simulink model "LTS_GGV"  (R2024b)
settings: Solver=ode4  StartTime=0.0  StopTime=5  FixedStep=0.001  RelTol=1e-3
values from neighbouring files (symbols this model uses):
  Accelcmd = 0    [generate_GGV_LTS_GGV.m]
  Decelcmd = Brk    [generate_GGV_LTS_GGV.m]
  Omega0 = V0/Rw    [generate_GGV_LTS_GGV.m]
  Steer_rad = deg2rad(SteerDeg)    [generate_GGV_LTS_GGV.m]
libraries: autolibsharedcoupling x1, vehdynlibsteering x1, autolibmappedmotor x1, autolibshared x1
(part 2 of 2)

== matlab function LTS_GGV/Rear_left tire  ==
  data: alpha input; Fx output; gamma input; kappa input; Fz input; Vc input; a input; b input; re input; mu0 input; cp input; n input; Fy output; Mz output; Mx output; slide_count output
function [Fx,Fy,Mz,Mx,slide_count] = tread_model( ...
                alpha,...
                gamma,...
                kappa,...
                Fz,...
                Vc,...
                a,b,re,...
                mu0,...
                cp,...
                n)

%%%%%%%%%%%%%%%%%%%%%%%%%%%%%%%%%%%%%%%%%%%%%%%%%%%%%%%%%%%%
% CONTACT PATCH
%%%%%%%%%%%%%%%%%%%%%%%%%%%%%%%%%%%%%%%%%%%%%%%%%%%%%%%%%%%%

xb = linspace(a,-a,n);

dx = abs(xb(2)-xb(1));

%%%%%%%%%%%%%%%%%%%%%%%%%%%%%%%%%%%%%%%%%%%%%%%%%%%%%%%%%%%%
% ROLLING KINEMATICS
%%%%%%%%%%%%%%%%%%%%%%%%%%%%%%%%%%%%%%%%%%%%%%%%%%%%%%%%%%%%

Vr = Vc/(1-kappa);

Omega = Vr/re;

dt = dx/Vr;

%%%%%%%%%%%%%%%%%%%%%%%%%%%%%%%%%%%%%%%%%%%%%%%%%%%%%%%%%%%%
% SLIP VELOCITIES
%%%%%%%%%%%%%%%%%%%%%%%%%%%%%%%%%%%%%%%%%%%%%%%%%%%%%%%%%%%%

Vsx = -Vc*kappa;

Vsy = -Vc*tan(alpha);

%%%%%%%%%%%%%%%%%%%%%%%%%%%%%%%%%%%%%%%%%%%%%%%%%%%%%%%%%%%%
% MULTI ROW TREAD
%%%%%%%%%%%%%%%%%%%%%%%%%%%%%%%%%%%%%%%%%%%%%%%%%%%%%%%%%%%%

nRows = 11;

yrow = linspace(-b,b,nRows);

dyrow = (2*b)/(nRows-1);

%%%%%%%%%%%%%%%%%%%%%%%%%%%%%%%%%%%%%%%%%%%%%%%%%%%%%%%%%%%%
% OUTPUT INITIALIZATION
%%%%%%%%%%%%%%%%%%%%%%%%%%%%%%%%%%%%%%%%%%%%%%%%%%%%%%%%%%%%

Fx = 0;
Fy = 0;
Mz = 0;
Mx = 0;

slide_count = 0;

%%%%%%%%%%%%%%%%%%%%%%%%%%%%%%%%%%%%%%%%%%%%%%%%%%%%%%%%%%%%
% PRESSURE NORMALIZATION
%%%%%%%%%%%%%%%%%%%%%%%%%%%%%%%%%%%%%%%%%%%%%%%%%%%%%%%%%%%%

ShapeSum = 0;

for r = 1:nRows

    yb0 = yrow(r);

    for i = 1:n

        px = max(0,1-(xb(i)/a)^2);

        py = sqrt(max(0,1-(yb0/b)^2));

        ShapeSum = ShapeSum + px*py*dx*dyrow;

    end
end

qz0 = Fz/ShapeSum;

%%%%%%%%%%%%%%%%%%%%%%%%%%%%%%%%%%%%%%%%%%%%%%%%%%%%%%%%%%%%
% MAIN LOOP
%%%%%%%%%%%%%%%%%%%%%%%%%%%%%%%%%%%%%%%%%%%%%%%%%%%%%%%%%%%%

for r = 1:nRows

    yb0 = yrow(r);

    ex = 0;
    ey = 0;

    for i = 1:n

        px = max(0,1-(xb(i)/a)^2);

        py = sqrt(max(0,1-(yb0/b)^2));

        qz = qz0*px*py;

        if qz <= 0
            continue
        end

        dybdx = (xb(i)/re)*sin(gamma);

        Vbx = Vsx + yb0*Omega*sin(gamma);

        Vby = Vsy - Vr*dybdx;

        %%%%%%%%%%%%%%%%%%%%%%%%%%%%%%%%%%%%%%%%%%%%%%%%%%%%
        % CONSTANT FRICTION
        %%%%%%%%%%%%%%%%%%%%%%%%%%%%%%%%%%%%%%%%%%%%%%%%%%%%

        qlimit = mu0*qz;

        Dsx = Vbx*dt;

        Dsy = Vby*dt;

        ex_trial = ex - Dsx;

        ey_trial = ey - Dsy;

        qx_trial = cp*ex_trial;

        qy_trial = cp*ey_trial;

        qtrial = hypot(qx_trial,qy_trial);

        %%%%%%%%%%%%%%%%%%%%%%%%%%%%%%%%%%%%%%%%%%%%%%%%%%%%
        % ADHESION
        %%%%%%%%%%%%%%%%%%%%%%%%%%%%%%%%%%%%%%%%%%%%%%%%%%%%

        if qtrial <= qlimit

            ex = ex_trial;
            ey = ey_trial;

            qx = cp*ex;
            qy = cp*ey;

        %%%%%%%%%%%%%%%%%%%%%%%%%%%%%%%%%%%%%%%%%%%%%%%%%%%%
        % SLIDING
        %%%%%%%%%%%%%%%%%%%%%%%%%%%%%%%%%%%%%%%%%%%%%%%%%%%%

        else

            slide_count = slide_count + 1;

            e_i = qlimit/cp;

            norm_trial = hypot(ex_trial,ey_trial);

            if norm_trial > 1e-12

                ex = e_i*ex_trial/norm_trial;

                ey = e_i*ey_trial/norm_trial;

            else

                ex = 0;
                ey = 0;

            end

            qx = cp*ex;
            qy = cp*ey;

        end

        dA = dx*dyrow;

        dFx = qx*dA;
        dFy = qy*dA;

        Fx = Fx + dFx;
        Fy = Fy + dFy;

        Mz = Mz + xb(i)*dFy - yb0*dFx;

        Mx = Mx + yb0*dFy;

    end
end

end

== matlab function LTS_GGV/Wheel kinematics ==
  data: Ux input; alphaFL output; Uy input; r input; deltaFL input; deltaFR input; omegaFL input; omegaFR input; omegaRL input; omegaRR input; lf input; lr input; tf input; tr input; Rw input; alphaFR output; alphaRL output; alphaRR output; kappaFL output; kappaFR output; kappaRL output; kappaRR output; VcFL output; VcFR output; VcRL output; VcRR output; VxwFL output; VywFL output; VxwFR output; VywFR output
function [alphaFL,alphaFR,alphaRL,alphaRR, ...
          kappaFL,kappaFR,kappaRL,kappaRR, ...
          VcFL,VcFR,VcRL,VcRR, ...
          VxwFL,VywFL,VxwFR,VywFR] = WheelKinematics( ...
          Ux,Uy,r, ...
          deltaFL,deltaFR, ...
          omegaFL,omegaFR,omegaRL,omegaRR, ...
          lf,lr,tf,tr,Rw)

%#codegen

%% =========================================================
% Numerical protection
% =========================================================

Veps = 0.5;

%% =========================================================
% Wheel-centre velocities in vehicle frame
%
% x = forward
% y = left
% r = positive CCW
% =========================================================

VxFL = Ux - r*tf/2;
VyFL = Uy + r*lf;

VxFR = Ux + r*tf/2;
VyFR = Uy + r*lf;

VxRL = Ux - r*tr/2;
VyRL = Uy - r*lr;

VxRR = Ux + r*tr/2;
VyRR = Uy - r*lr;

%% =========================================================
% Transform front-wheel velocities into wheel coordinates
% =========================================================

cFL = cos(deltaFL);
sFL = sin(deltaFL);

cFR = cos(deltaFR);
sFR = sin(deltaFR);

VxwFL =  VxFL*cFL + VyFL*sFL;
VywFL = -VxFL*sFL + VyFL*cFL;

VxwFR =  VxFR*cFR + VyFR*sFR;
VywFR = -VxFR*sFR + VyFR*cFR;

%% =========================================================
% Rear wheels are not steered
% =========================================================

VxwRL = VxRL;
VywRL = VyRL;

VxwRR = VxRR;
VywRR = VyRR;

%% =========================================================
% Slip angles
%
% Tire model convention:
% positive alpha -> positive Fy
% =========================================================

alphaFL = -atan2(VywFL, max(abs(VxwFL),Veps));
alphaFR = -atan2(VywFR, max(abs(VxwFR),Veps));

alphaRL = -atan2(VywRL, max(abs(VxwRL),Veps));
alphaRR = -atan2(VywRR, max(abs(VxwRR),Veps));

%% =========================================================
% Longitudinal contact velocity
% =========================================================

VcFL = max(abs(VxwFL),Veps);
VcFR = max(abs(VxwFR),Veps);

VcRL = max(abs(VxwRL),Veps);
VcRR = max(abs(VxwRR),Veps);

%% =========================================================
% Slip ratio
%
% Positive kappa = driving
% Negative kappa = braking
%
% IMPORTANT:
% Do NOT artificially saturate kappa here.
% The tire model should impose the physical friction limit.
% =========================================================

kappaFL = (Rw*omegaFL - VxwFL) / VcFL;
kappaFR = (Rw*omegaFR - VxwFR) / VcFR;

kappaRL = (Rw*omegaRL - VxwRL) / VcRL;
kappaRR = (Rw*omegaRR - VxwRR) / VcRR;

end

== matlab function LTS_GGV/Front_Left_tire ==
  data: alpha input; Fx output; gamma input; kappa input; Fz input; Vc input; a input; b input; re input; mu0 input; cp input; n input; Fy output; Mz output; Mx output; slide_count output
function [Fx,Fy,Mz,Mx,slide_count] = tread_model( ...
                alpha,...
                gamma,...
                kappa,...
                Fz,...
                Vc,...
                a,b,re,...
                mu0,...
                cp,...
                n)

%%%%%%%%%%%%%%%%%%%%%%%%%%%%%%%%%%%%%%%%%%%%%%%%%%%%%%%%%%%%
% CONTACT PATCH
%%%%%%%%%%%%%%%%%%%%%%%%%%%%%%%%%%%%%%%%%%%%%%%%%%%%%%%%%%%%

xb = linspace(a,-a,n);

dx = abs(xb(2)-xb(1));

%%%%%%%%%%%%%%%%%%%%%%%%%%%%%%%%%%%%%%%%%%%%%%%%%%%%%%%%%%%%
% ROLLING KINEMATICS
%%%%%%%%%%%%%%%%%%%%%%%%%%%%%%%%%%%%%%%%%%%%%%%%%%%%%%%%%%%%

Vr = Vc/(1-kappa);

Omega = Vr/re;

dt = dx/Vr;

%%%%%%%%%%%%%%%%%%%%%%%%%%%%%%%%%%%%%%%%%%%%%%%%%%%%%%%%%%%%
% SLIP VELOCITIES
%%%%%%%%%%%%%%%%%%%%%%%%%%%%%%%%%%%%%%%%%%%%%%%%%%%%%%%%%%%%

Vsx = -Vc*kappa;

Vsy = -Vc*tan(alpha);

%%%%%%%%%%%%%%%%%%%%%%%%%%%%%%%%%%%%%%%%%%%%%%%%%%%%%%%%%%%%
% MULTI ROW TREAD
%%%%%%%%%%%%%%%%%%%%%%%%%%%%%%%%%%%%%%%%%%%%%%%%%%%%%%%%%%%%

nRows = 11;

yrow = linspace(-b,b,nRows);

dyrow = (2*b)/(nRows-1);

%%%%%%%%%%%%%%%%%%%%%%%%%%%%%%%%%%%%%%%%%%%%%%%%%%%%%%%%%%%%
% OUTPUT INITIALIZATION
%%%%%%%%%%%%%%%%%%%%%%%%%%%%%%%%%%%%%%%%%%%%%%%%%%%%%%%%%%%%

Fx = 0;
Fy = 0;
Mz = 0;
Mx = 0;

slide_count = 0;

%%%%%%%%%%%%%%%%%%%%%%%%%%%%%%%%%%%%%%%%%%%%%%%%%%%%%%%%%%%%
% PRESSURE NORMALIZATION
%%%%%%%%%%%%%%%%%%%%%%%%%%%%%%%%%%%%%%%%%%%%%%%%%%%%%%%%%%%%

ShapeSum = 0;

for r = 1:nRows

    yb0 = yrow(r);

    for i = 1:n

        px = max(0,1-(xb(i)/a)^2);

        py = sqrt(max(0,1-(yb0/b)^2));

        ShapeSum = ShapeSum + px*py*dx*dyrow;

    end
end

qz0 = Fz/ShapeSum;

%%%%%%%%%%%%%%%%%%%%%%%%%%%%%%%%%%%%%%%%%%%%%%%%%%%%%%%%%%%%
% MAIN LOOP
%%%%%%%%%%%%%%%%%%%%%%%%%%%%%%%%%%%%%%%%%%%%%%%%%%%%%%%%%%%%

for r = 1:nRows

    yb0 = yrow(r);

    ex = 0;
    ey = 0;

    for i = 1:n

        px = max(0,1-(xb(i)/a)^2);

        py = sqrt(max(0,1-(yb0/b)^2));

        qz = qz0*px*py;

        if qz <= 0
            continue
        end

        dybdx = (xb(i)/re)*sin(gamma);

        Vbx = Vsx + yb0*Omega*sin(gamma);

        Vby = Vsy - Vr*dybdx;

        %%%%%%%%%%%%%%%%%%%%%%%%%%%%%%%%%%%%%%%%%%%%%%%%%%%%
        % CONSTANT FRICTION
        %%%%%%%%%%%%%%%%%%%%%%%%%%%%%%%%%%%%%%%%%%%%%%%%%%%%

        qlimit = mu0*qz;

        Dsx = Vbx*dt;

        Dsy = Vby*dt;

        ex_trial = ex - Dsx;

        ey_trial = ey - Dsy;

        qx_trial = cp*ex_trial;

        qy_trial = cp*ey_trial;

        qtrial = hypot(qx_trial,qy_trial);

        %%%%%%%%%%%%%%%%%%%%%%%%%%%%%%%%%%%%%%%%%%%%%%%%%%%%
        % ADHESION
        %%%%%%%%%%%%%%%%%%%%%%%%%%%%%%%%%%%%%%%%%%%%%%%%%%%%

        if qtrial <= qlimit

            ex = ex_trial;
            ey = ey_trial;

            qx = cp*ex;
            qy = cp*ey;

        %%%%%%%%%%%%%%%%%%%%%%%%%%%%%%%%%%%%%%%%%%%%%%%%%%%%
        % SLIDING
        %%%%%%%%%%%%%%%%%%%%%%%%%%%%%%%%%%%%%%%%%%%%%%%%%%%%

        else

            slide_count = slide_count + 1;

            e_i = qlimit/cp;

            norm_trial = hypot(ex_trial,ey_trial);

            if norm_trial > 1e-12

                ex = e_i*ex_trial/norm_trial;

                ey = e_i*ey_trial/norm_trial;

            else

                ex = 0;
                ey = 0;

            end

            qx = cp*ex;
            qy = cp*ey;

        end

        dA = dx*dyrow;

        dFx = qx*dA;
        dFy = qy*dA;

        Fx = Fx + dFx;
        Fy = Fy + dFy;

        Mz = Mz + xb(i)*dFy - yb0*dFx;

        Mx = Mx + yb0*dFy;

    end
end

end
